simulink model "House_model"  (R2016b)
settings: Solver=VariableStepAuto  StartTime=0.0  StopTime=inf  RelTol=1e-3
settings Model: Creator=isabelle  LastModifiedBy=isabelle

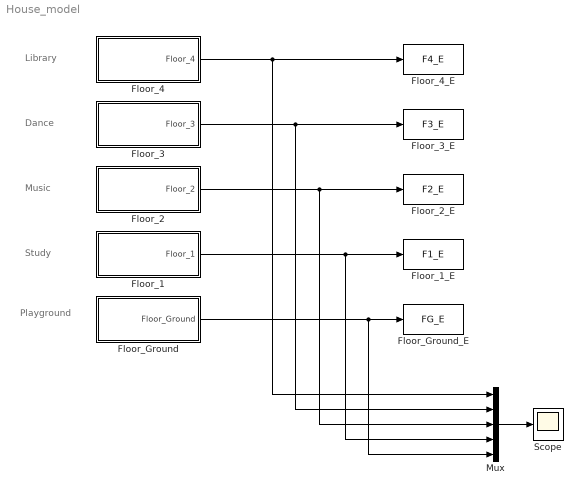
== system House_model ==
  note: Library
  note: Dance
  note: Music
  note: Study
  note: Playground
  Floor_1 : Subsystem
  Floor_1_E : ToWorkspace  VariableName=F1_E  SaveFormat=Timeseries  SampleTime=-1
  Floor_2 : Subsystem
  Floor_2_E : ToWorkspace  VariableName=F2_E  SaveFormat=Timeseries  SampleTime=-1
  Floor_3 : Subsystem
  Floor_3_E : ToWorkspace  VariableName=F3_E  SaveFormat=Timeseries  SampleTime=-1
  Floor_4 : Subsystem
  Floor_4_E : ToWorkspace  VariableName=F4_E  SaveFormat=Timeseries  SampleTime=-1
  Floor_Ground : Subsystem
  Floor_Ground_E : ToWorkspace  VariableName=FG_E  SaveFormat=Timeseries  SampleTime=-1
  Mux : Mux  Inputs=5
  Scope : Scope
  wires:
  Floor_4/1(Floor_4) -> Mux/1, Floor_4_E/1
  Floor_3/1(Floor_3) -> Mux/2, Floor_3_E/1
  Floor_Ground/1(Floor_Ground) -> Mux/5, Floor_Ground_E/1
  Floor_1/1(Floor_1) -> Mux/4, Floor_1_E/1
  Floor_2/1(Floor_2) -> Mux/3, Floor_2_E/1
  Mux/1 -> Scope/1

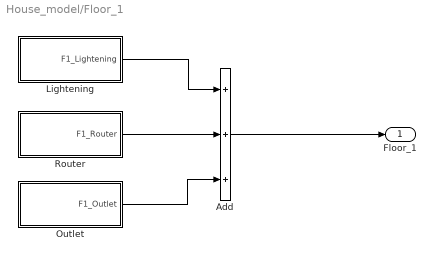
== system House_model/Floor_1 ==
  Add : Sum  Inputs=3
  Lightening : Subsystem
  Outlet : Subsystem
  Router : Subsystem
  Floor_1 : Outport
  wires:
  Lightening/1(F1_Lightening) -> Add/1
  Router/1(F1_Router) -> Add/2
  Outlet/1(F1_Outlet) -> Add/3
  Add/1 -> Floor_1/1

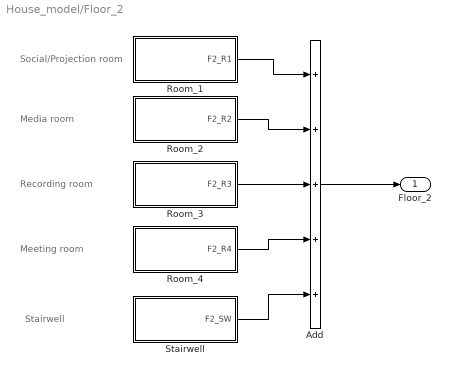
== system House_model/Floor_2 ==
  note: Social/Projection room
  note: Media room
  note: Recording room
  note: Meeting room
  note: Stairwell
  Add : Sum  Inputs=5
  Room_1 : Subsystem
  Room_2 : Subsystem
  Room_3 : Subsystem
  Room_4 : Subsystem
  Stairwell : Subsystem
  Floor_2 : Outport
  wires:
  Add/1 -> Floor_2/1
  Room_1/1(F2_R1) -> Add/1
  Room_2/1(F2_R2) -> Add/2
  Room_3/1(F2_R3) -> Add/3
  Stairwell/1(F2_SW) -> Add/5
  Room_4/1(F2_R4) -> Add/4

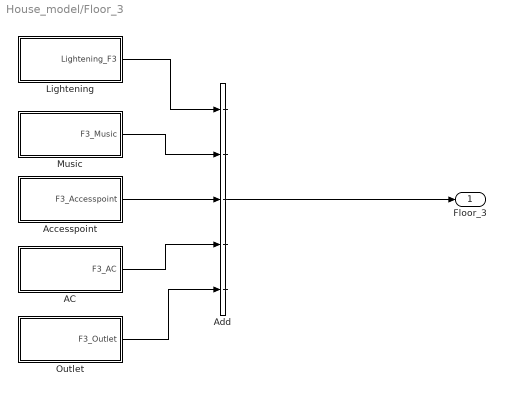
== system House_model/Floor_3 ==
  AC : Subsystem
  Accesspoint : Subsystem
  Add : Sum  Inputs=5
  Lightening : Subsystem
  Music : Subsystem
  Outlet : Subsystem
  Floor_3 : Outport
  wires:
  Lightening/1(Lightening_F3) -> Add/1
  Outlet/1(F3_Outlet) -> Add/5
  Music/1(F3_Music) -> Add/2
  Accesspoint/1(F3_Accesspoint) -> Add/3
  AC/1(F3_AC) -> Add/4
  Add/1 -> Floor_3/1

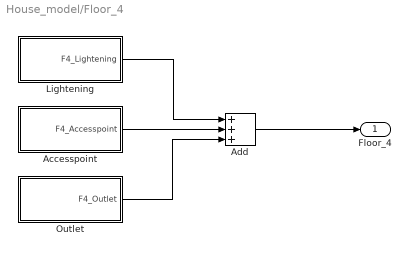
== system House_model/Floor_4 ==
  Accesspoint : Subsystem
  Add : Sum  Inputs=3
  Lightening : Subsystem
  Outlet : Subsystem
  Floor_4 : Outport
  wires:
  Lightening/1(F4_Lightening) -> Add/1
  Accesspoint/1("F4_Accesspoint ") -> Add/2
  Add/1 -> Floor_4/1
  Outlet/1("F4_Outlet ") -> Add/3

== system House_model/Floor_Ground ==
  Lightening : Subsystem
  Floor_Ground : Outport
  wires:
  Lightening/1(FG_Lightening) -> Floor_Ground/1

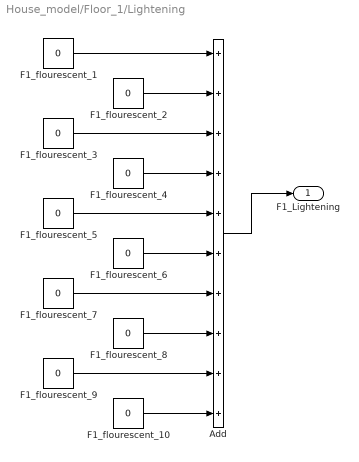
== system House_model/Floor_1/Lightening ==
  Add : Sum  Inputs=10
  F1_flourescent_{1..10} (10 alike) : Constant  Value=0
  F1_Lightening : Outport
  wires:
  F1_flourescent_1/1 -> Add/1
  F1_flourescent_2/1 -> Add/2
  Add/1 -> F1_Lightening/1
  F1_flourescent_3/1 -> Add/3
  F1_flourescent_4/1 -> Add/4
  F1_flourescent_5/1 -> Add/5
  F1_flourescent_6/1 -> Add/6
  F1_flourescent_7/1 -> Add/7
  F1_flourescent_8/1 -> Add/8
  F1_flourescent_9/1 -> Add/9
  F1_flourescent_10/1 -> Add/10

== system House_model/Floor_1/Outlet ==
  Add : Sum  Inputs=2
  F1_laptops : Constant  Value=0
  F1_phones : Constant  Value=0
  F1_Outlet : Outport
  wires:
  F1_phones/1 -> Add/1
  F1_laptops/1 -> Add/2
  Add/1 -> F1_Outlet/1

== system House_model/Floor_1/Router ==
  F1_router : Constant  Value=0
  F1_Router : Outport
  wires:
  F1_router/1 -> F1_Router/1

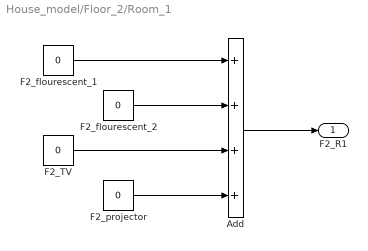
== system House_model/Floor_2/Room_1 ==
  Add : Sum  Inputs=4
  F2_TV : Constant  Value=0
  F2_flourescent_1 : Constant  Value=0
  F2_flourescent_2 : Constant  Value=0
  F2_projector : Constant  Value=0
  F2_R1 : Outport
  wires:
  Add/1 -> F2_R1/1
  F2_flourescent_1/1 -> Add/1
  F2_flourescent_2/1 -> Add/2
  F2_TV/1 -> Add/3
  F2_projector/1 -> Add/4

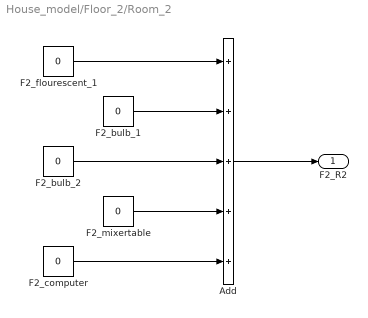
== system House_model/Floor_2/Room_2 ==
  Add : Sum  Inputs=5
  F2_bulb_1 : Constant  Value=0
  F2_bulb_2 : Constant  Value=0
  F2_computer : Constant  Value=0
  F2_flourescent_1 : Constant  Value=0
  F2_mixertable : Constant  Value=0
  F2_R2 : Outport
  wires:
  F2_flourescent_1/1 -> Add/1
  F2_bulb_1/1 -> Add/2
  Add/1 -> F2_R2/1
  F2_mixertable/1 -> Add/4
  F2_computer/1 -> Add/5
  F2_bulb_2/1 -> Add/3

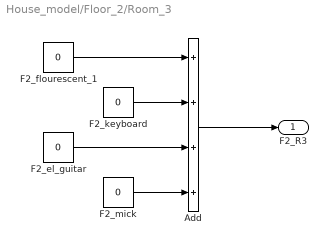
== system House_model/Floor_2/Room_3 ==
  Add : Sum  Inputs=4
  F2_el_guitar : Constant  Value=0
  F2_flourescent_1 : Constant  Value=0
  F2_keyboard : Constant  Value=0
  F2_mick : Constant  Value=0
  F2_R3 : Outport
  wires:
  F2_flourescent_1/1 -> Add/1
  F2_keyboard/1 -> Add/2
  Add/1 -> F2_R3/1
  F2_el_guitar/1 -> Add/3
  F2_mick/1 -> Add/4

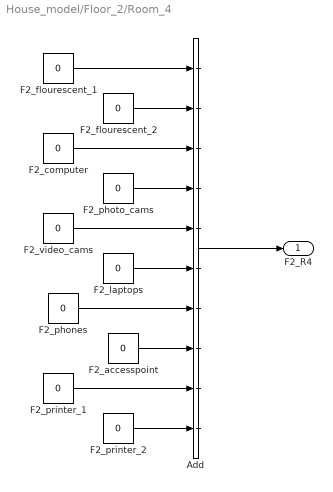
== system House_model/Floor_2/Room_4 ==
  Add : Sum  Inputs=10
  F2_accesspoint : Constant  Value=0
  F2_computer : Constant  Value=0
  F2_flourescent_1 : Constant  Value=0
  F2_flourescent_2 : Constant  Value=0
  F2_laptops : Constant  Value=0
  F2_phones : Constant  Value=0
  F2_photo_cams : Constant  Value=0
  F2_printer_1 : Constant  Value=0
  F2_printer_2 : Constant  Value=0
  F2_video_cams : Constant  Value=0
  F2_R4 : Outport
  wires:
  F2_flourescent_1/1 -> Add/1
  F2_flourescent_2/1 -> Add/2
  Add/1 -> F2_R4/1
  F2_computer/1 -> Add/3
  F2_photo_cams/1 -> Add/4
  F2_video_cams/1 -> Add/5
  F2_laptops/1 -> Add/6
  F2_phones/1 -> Add/7
  F2_accesspoint/1 -> Add/8
  F2_printer_1/1 -> Add/9
  F2_printer_2/1 -> Add/10

== system House_model/Floor_2/Stairwell ==
  Add : Sum  Inputs=2
  F2_bulb_1 : Constant  Value=0
  F2_flourescent_1 : Constant  Value=0
  F2_SW : Outport
  wires:
  F2_flourescent_1/1 -> Add/1
  F2_bulb_1/1 -> Add/2
  Add/1 -> F2_SW/1

== system House_model/Floor_3/AC ==
  F3_AC_1 : Constant  Value=0
  F3_AC : Outport
  wires:
  F3_AC_1/1 -> F3_AC/1

== system House_model/Floor_3/Accesspoint ==
  F3_accesspoint_1 : Constant  Value=0
  F3_Accesspoint : Outport
  wires:
  F3_accesspoint_1/1 -> F3_Accesspoint/1

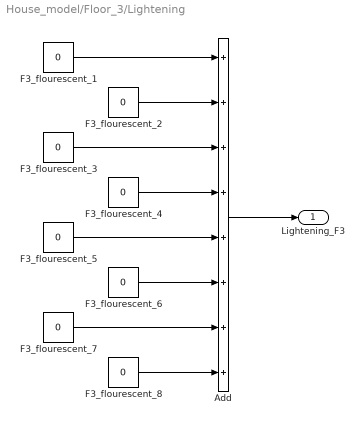
== system House_model/Floor_3/Lightening ==
  Add : Sum  Inputs=8
  F3_flourescent_{1..8} (8 alike) : Constant  Value=0
  Lightening_F3 : Outport
  wires:
  F3_flourescent_1/1 -> Add/1
  F3_flourescent_2/1 -> Add/2
  F3_flourescent_3/1 -> Add/3
  F3_flourescent_4/1 -> Add/4
  F3_flourescent_5/1 -> Add/5
  F3_flourescent_6/1 -> Add/6
  Add/1 -> Lightening_F3/1
  F3_flourescent_7/1 -> Add/7
  F3_flourescent_8/1 -> Add/8

== system House_model/Floor_3/Music ==
  Add : Sum  Inputs=3
  F3_reciver : Constant  Value=0
  F3_speakers : Constant  Value=0
  F3_subwoofer : Constant  Value=0
  F3_Music : Outport
  wires:
  F3_subwoofer/1 -> Add/1
  F3_reciver/1 -> Add/2
  F3_speakers/1 -> Add/3
  Add/1 -> F3_Music/1

== system House_model/Floor_3/Outlet ==
  Add : Sum  Inputs=2
  F3_Laptops : Constant  Value=0
  F3_Phones : Constant  Value=0
  F3_Outlet : Outport
  wires:
  F3_Phones/1 -> Add/1
  F3_Laptops/1 -> Add/2
  Add/1 -> F3_Outlet/1

== system House_model/Floor_4/Accesspoint ==
  F4_Accesspoint : Constant  Value=6.5
  "F4_Accesspoint " : Outport
  wires:
  F4_Accesspoint/1 -> "F4_Accesspoint "/1

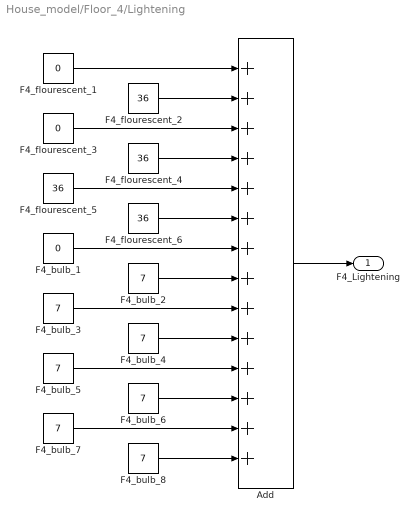
== system House_model/Floor_4/Lightening ==
  Add : Sum  Inputs=14
  F4_bulb_1 : Constant  Value=0
  F4_bulb_{2..8} (7 alike) : Constant  Value=7
  F4_flourescent_1 : Constant  Value=0
  F4_flourescent_{2,4..6} (4 alike) : Constant  Value=36
  F4_flourescent_3 : Constant  Value=0
  F4_Lightening : Outport
  wires:
  F4_flourescent_1/1 -> Add/1
  F4_flourescent_2/1 -> Add/2
  F4_flourescent_3/1 -> Add/3
  F4_flourescent_4/1 -> Add/4
  F4_flourescent_5/1 -> Add/5
  F4_bulb_1/1 -> Add/7
  F4_bulb_2/1 -> Add/8
  F4_bulb_3/1 -> Add/9
  F4_bulb_4/1 -> Add/10
  F4_bulb_5/1 -> Add/11
  F4_flourescent_6/1 -> Add/6
  F4_bulb_7/1 -> Add/13
  F4_bulb_8/1 -> Add/14
  F4_bulb_6/1 -> Add/12
  Add/1 -> F4_Lightening/1

== system House_model/Floor_4/Outlet ==
  Add : Sum
  F4_Laptops : Constant  Value=270
  F4_Phones : Constant  Value=270
  "F4_Outlet " : Outport
  wires:
  F4_Phones/1 -> Add/1
  Add/1 -> "F4_Outlet "/1
  F4_Laptops/1 -> Add/2

== system House_model/Floor_Ground/Lightening ==
  Add : Sum
  FG_flourescent_1 : Constant  Value=0
  FG_flourescent_2 : Constant  Value=0
  FG_Lightening : Outport
  wires:
  FG_flourescent_1/1 -> Add/1
  FG_flourescent_2/1 -> Add/2
  Add/1 -> FG_Lightening/1
